simulink model "KF_Template"  (R2015b)
settings: Solver=VariableStepAuto  StartTime=0.0  StopTime=10.0  RelTol=1e-3
values from neighbouring files (symbols this model uses):
  dT = quadEDT.sampletime    [parameters_estimationcontrol.m]
  sigmaW = blkdiag(0.001, 10)    [parameters_estimationcontrol.m]
  sigmaX0 = zeros(2,2)    [parameters_estimationcontrol.m]
  x0 = [-0.046 0]    [parameters_estimationcontrol.m]
settings Model: Creator=student  LastModifiedBy=student

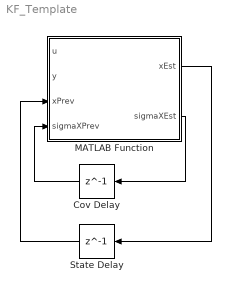
== system KF_Template ==
  Cov Delay : Delay  DelayLength=1  InitialCondition=sigmaX0
  MATLAB Function : MATLAB Function  TreatAsAtomicUnit=on
  State Delay : Delay  DelayLength=1  InitialCondition=x0
  wires:
  MATLAB Function/2(sigmaXEst) -> Cov Delay/1
  Cov Delay/1 -> MATLAB Function/4(sigmaXPrev)
  MATLAB Function/1(xEst) -> State Delay/1
  State Delay/1 -> MATLAB Function/3(xPrev)

== matlab function KF_Template/MATLAB Function ==
  data: u input; xEst output; y input; xPrev input; sigmaXPrev input; sigmaW parameter; dT parameter; sigmaXEst output
function [xEst, sigmaXEst] = KalmanFilter(u, y, xPrev, sigmaXPrev, sigmaW, dT)
%#codegen
% This function implements the discrete time invariant Kalman Filter
%
% Inputs:
%           u - system input
%           y - output measurement
%           xPrev - state estimate at previous time step
%           sigmaXPrev - state covariance estiamte at previous time step
%           sigmaW - noise covariance
%           dT - sampling time
%
% Outputs:
%           xEst - state estimate
%           sigmaXEst - state covariance estimate


% Define System Dynamics
% x(k+1) = A*x(k) + B*u(k) + E*w(k)
% y(k) = C*x(k) + F*w(k)

A = [1 dT; 0 1];
B = [0; dT];
E = [0 0; dT 0];
C = [1 0];
F = [0 1];

% Implement Kalman Filter
sigmaY_kk1 = C*sigmaXPrev*C' + F*sigmaW*F';
sigmaX_kk = sigmaXPrev - sigmaXPrev*C'/(sigmaY_kk1)*C*sigmaXPrev;
sigmaXEst = A*sigmaX_kk*A' + E*sigmaW*E';
e_k = y - C*xPrev;
x_kk = xPrev + sigmaXPrev*C'/(sigmaY_kk1)*(e_k);
xEst = A*x_kk + B*u;
